simulink model "physical_system"  (R2026a)
settings: Solver=VariableStepAuto
libraries: simulink x1
settings Model: Creator=tanmay  LastModifiedBy=tanmay

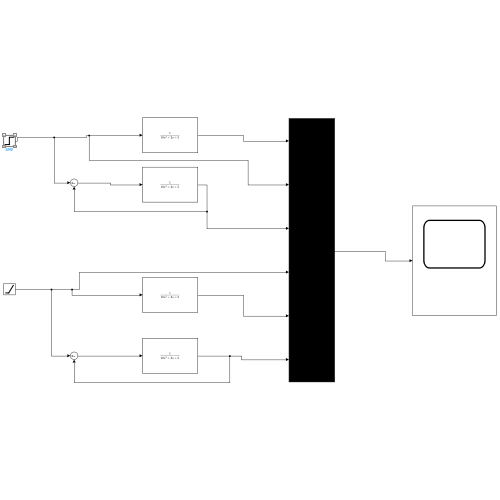
[thumbnail: Simulink's stored preview of the top-level diagram]
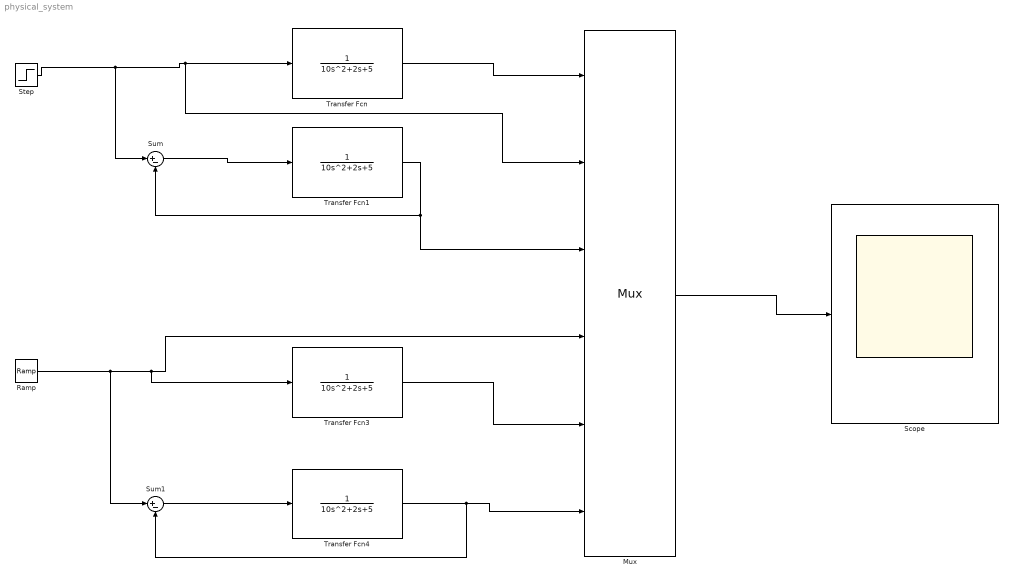
== system physical_system ==
  Mux : Mux  Inputs=6
  Ramp : simulink/Sources/Ramp  slope=1  start=0  InitialOutput=0
  Scope : Scope
      settings: ActiveDisplayYMinimum=-1.2499999999999998  ActiveDisplayYMaximum=11.25
  Step : Step  SampleTime=0
  Sum : Sum  Inputs=|+-
  Sum1 : Sum  Inputs=|+-
  Transfer Fcn{,1,3..4} (4 alike) : TransferFcn  Denominator=[10 2 5]
  wires:
  Step/1 -> Sum/1, Mux/2, Transfer Fcn/1
  Sum/1 -> Transfer Fcn1/1
  Transfer Fcn1/1 -> Mux/3, Sum/2
  Transfer Fcn/1 -> Mux/1
  Ramp/1 -> Sum1/1, Transfer Fcn3/1, Mux/4
  Transfer Fcn3/1 -> Mux/5
  Transfer Fcn4/1 -> Sum1/2, Mux/6
  Sum1/1 -> Transfer Fcn4/1
  Mux/1 -> Scope/1
